simulink model "sampleModel1722_2"  (R2023a)
settings: Solver=VariableStepAuto  StartTime=0.0  StopTime=10.0  RelTol=1e-3
libraries: hdlsllib x5, simulink x1
settings Model: Creator=user1  LastModifiedBy=user1

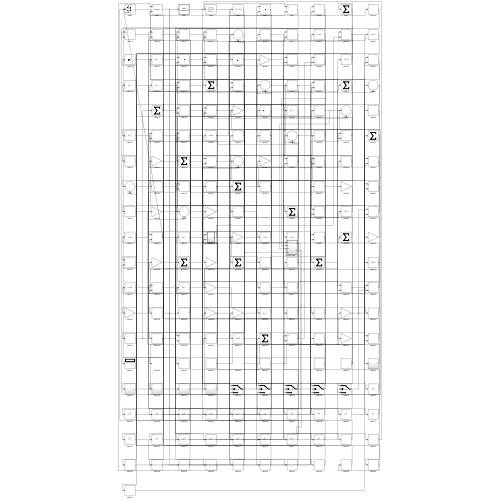
[thumbnail: Simulink's stored preview of the top-level diagram]
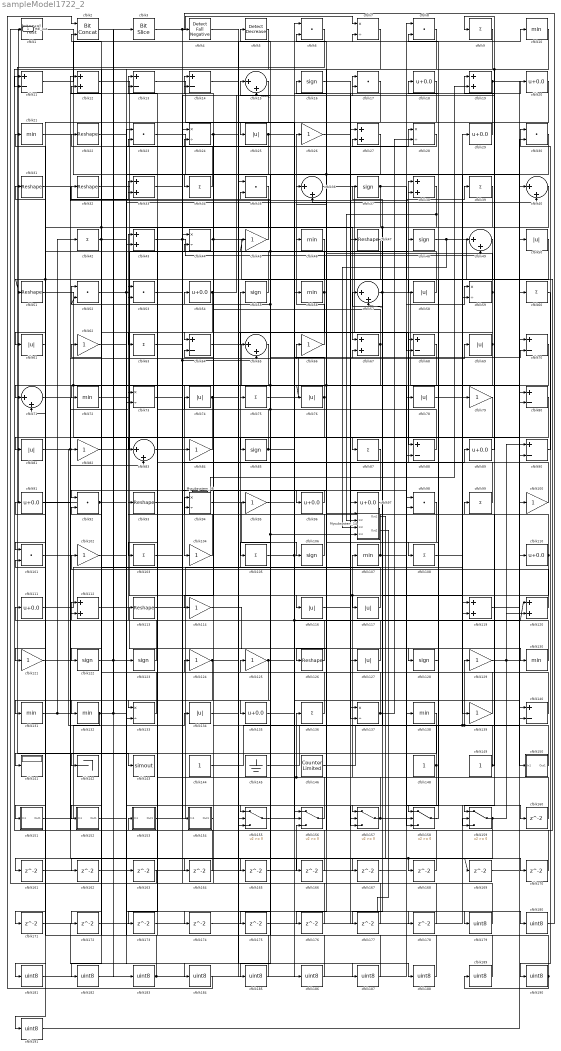
== system sampleModel1722_2 ==
  Mysubsystem_14 : Subsystem  TreatAsAtomicUnit=on  RTWFcnName=Mysubsystem_14
      settings: RTWFcnNameOpts=User specified  RTWFileNameOpts=Use function name
  Mysubsystem_36 : Subsystem  TreatAsAtomicUnit=on  RTWFcnName=Mysubsystem_36
      settings: RTWFcnNameOpts=User specified  RTWFileNameOpts=Use function name
  cfblk1 : hdlsllib/Logic and Bit Operations/Interval Test  IntervalClosedRight=on  uplimit=0.5  IntervalClosedLeft=on  lowlimit=-0.5  OutDataTypeStr=uint8
  cfblk{10,21,46,56,72,107,130..132,138} (10 alike) : MinMax  OutDataTypeStr=uint8
  cfblk{26,45,62,66,79,82,84,95,100,102,104,114,121,124..125,129,139} (17 alike) : Gain  OutDataTypeStr=uint8
  cfblk{6,8,17,23,30,35,52..53,92,98,101} (11 alike) : DotProduct  OutDataTypeStr=uint8
  cfblk{9,34,39,42,60,63,75,87,99,103,105,108,136} (13 alike) : Sum  Inputs=+  OutDataTypeStr=uint8
  cfblk{16,37,48,55,85,106,122..123,128} (9 alike) : Signum
  cfblk{11,13..14,64,68,70,80,88,90,140} (10 alike) : Sum  Inputs=+-  OutDataTypeStr=uint8
  cfblk{18,20,29,54,89,91,96..97,110..111,135} (11 alike) : Bias  Bias=0.0  SaturateOnIntegerOverflow=off
  cfblk{12,19,27,33,38,43,67,112,119..120} (10 alike) : Sum  OutDataTypeStr=uint8
  cfblk{22,31..32,47,51,93,113,126} (8 alike) : Reshape
  cfblk{25,50,58,61,69,74,76,78,81,116..117,127,134} (13 alike) : Abs  OutDataTypeStr=uint8  SaturateOnIntegerOverflow=off
  cfblk{7,24,28,44,59,73,94,133,137} (9 alike) : Product  Inputs=*/  OutDataTypeStr=uint8  RndMeth=Zero  SaturateOnIntegerOverflow=on
  cfblk141 : Display
  cfblk142 : Terminator
  cfblk143 : ToWorkspace  VariableName=simout  SaveFormat=Timeseries  SampleTime=-1
  cfblk144 : Constant  OutDataTypeStr=uint8  SampleTime=-1
  cfblk145 : Ground
  cfblk146 : hdlsllib/Sources/Counter Limited  uplimit=7  tsamp=-1
  cfblk148 : Constant  OutDataTypeStr=uint8  SampleTime=-1
  cfblk149 : Constant  OutDataTypeStr=uint8  SampleTime=-1
  cfblk{15,36,40,49,57,65,71,83} (8 alike) : Sum  Inputs=|++  OutDataTypeStr=uint8
  cfblk150 : Subsystem
      settings: LibrarySourceBlock=|
      | hdlsllib/Ports &
      | Subsystems/Subsystem
  cfblk151 : Subsystem
      settings: LibrarySourceBlock=|
      | hdlsllib/Ports &
      | Subsystems/Subsystem
  cfblk152 : Subsystem
      settings: LibrarySourceBlock=|
      | hdlsllib/Ports &
      | Subsystems/Subsystem
  cfblk153 : Subsystem
      settings: LibrarySourceBlock=|
      | hdlsllib/Ports &
      | Subsystems/Subsystem
  cfblk154 : Subsystem
      settings: LibrarySourceBlock=|
      | hdlsllib/Ports &
      | Subsystems/Subsystem
  cfblk{155..159} (5 alike) : Switch  OutDataTypeStr=uint8  SaturateOnIntegerOverflow=off  InputSameDT=off
  cfblk{160..178} (19 alike) : Delay  SampleTime=1
  cfblk{179..191} (13 alike) : DataTypeConversion  OutDataTypeStr=uint8  SaturateOnIntegerOverflow=off  RndMeth=Floor
  cfblk2 : hdlsllib/Logic and Bit Operations/Bit Concat  numInputs=2
  cfblk3 : hdlsllib/Logic and Bit Operations/Bit Slice  lidx=7  ridx=0
  cfblk4 : hdlsllib/Logic and Bit Operations/Detect Fall Negative  vinit=0  OutDataTypeStr=uint8
  cfblk5 : simulink/Logic and Bit Operations/Detect Decrease  vinit=0.0  OutDataTypeStr=uint8
      settings: LibrarySourceBlock=|
      | hdlsllib/Logic and Bit
      | Operations/Detect
      | Decrease
  Hdl_out : Outport  OutDataTypeStr=uint8
  wires:
  cfblk131/1 -> cfblk42/1, cfblk33/2
  cfblk100/1 -> cfblk38/1
  cfblk9/1 -> cfblk132/1
  cfblk132/1 -> cfblk3/1, cfblk159/3, cfblk82/1
  cfblk6/1 -> cfblk143/1
  cfblk66/1 -> cfblk26/1
  cfblk65/1 -> cfblk104/1
  cfblk157/1 -> cfblk107/1, cfblk39/1
  cfblk120/1 -> cfblk102/1
  cfblk12/1 -> cfblk116/1
  cfblk122/1 -> cfblk163/1, cfblk180/1
  cfblk113/1 -> cfblk55/1
  cfblk96/1 -> cfblk92/1
  cfblk103/1 -> cfblk117/1, cfblk119/2
  cfblk54/1 -> cfblk9/1, cfblk142/1
  cfblk98/1 -> cfblk126/1
  cfblk159/1 -> cfblk90/1, cfblk191/1
  cfblk107/1 -> cfblk75/1, cfblk59/1
  cfblk25/1 -> cfblk34/1, cfblk58/1
  cfblk133/1 -> cfblk92/2
  cfblk111/1 -> cfblk84/1
  cfblk123/1 -> cfblk43/1
  cfblk2/1 -> cfblk183/1
  cfblk32/1 -> cfblk67/1
  cfblk48/1 -> Mysubsystem_14/3(In3), cfblk153/1(In1)
  cfblk39/1 -> cfblk103/1, cfblk57/2
  cfblk117/1 -> cfblk52/1
  cfblk51/1 -> cfblk87/1, cfblk97/1
  cfblk112/1 -> cfblk130/1
  cfblk44/1 -> cfblk150/1(In1), cfblk14/1
  cfblk74/1 -> cfblk7/2, cfblk182/1
  cfblk85/1 -> cfblk74/1, cfblk157/3
  cfblk130/1 -> cfblk46/1
  cfblk19/1 -> cfblk140/1, cfblk81/1
  cfblk69/1 -> cfblk101/1, cfblk63/1
  cfblk42/1 -> cfblk28/1, cfblk12/2
  cfblk30/1 -> cfblk85/1
  cfblk153/1(Out1) -> cfblk29/1
  cfblk68/1 -> cfblk76/1, cfblk166/1
  cfblk47/1 -> cfblk133/1
  cfblk36/1 -> cfblk88/1
  cfblk145/1 -> cfblk129/1, cfblk90/2, cfblk79/1
  cfblk126/1 -> cfblk111/1
  cfblk92/1 -> cfblk123/1, Hdl_out/1
  cfblk27/1 -> Mysubsystem_14/1(In1), cfblk133/2
  cfblk99/1 -> cfblk32/1
  cfblk79/1 -> cfblk158/1
  cfblk83/1 -> cfblk66/1
  cfblk13/1 -> cfblk156/1
  cfblk82/1 -> cfblk48/1
  cfblk91/1 -> cfblk69/1
  cfblk140/1 -> cfblk13/1
  cfblk97/1 -> cfblk37/1
  cfblk11/1 -> cfblk10/1
  cfblk49/1 -> cfblk108/1
  cfblk20/1 -> cfblk122/1
  cfblk106/1 -> cfblk5/1
  cfblk110/1 -> cfblk93/1, cfblk167/1
  cfblk15/1 -> cfblk51/1, cfblk151/1(In1)
  cfblk35/1 -> cfblk171/1, cfblk172/1
  cfblk73/1 -> cfblk17/1, cfblk65/2
  cfblk67/1 -> cfblk72/1, cfblk24/2
  cfblk139/1 -> cfblk112/1
  cfblk144/1 -> cfblk78/1
  cfblk108/1 -> cfblk119/1
  cfblk56/1 -> cfblk64/1, cfblk35/2
  cfblk37/1 -> cfblk135/1, cfblk59/2
  cfblk146/1 -> cfblk40/1
  cfblk29/1 -> cfblk25/1
  cfblk137/1 -> cfblk54/1, cfblk28/2
  cfblk81/1 -> cfblk168/1, cfblk169/1, cfblk14/2
  cfblk116/1 -> cfblk20/1
  cfblk128/1 -> cfblk18/1
  cfblk78/1 -> cfblk49/1
  cfblk72/1 -> cfblk6/1
  cfblk31/1 -> cfblk38/2
  cfblk23/1 -> cfblk80/1
  cfblk84/1 -> cfblk83/1
  cfblk57/1 -> cfblk100/1, cfblk177/1
  cfblk59/1 -> cfblk6/2, cfblk176/1
  cfblk94/1 -> cfblk106/1
  cfblk33/1 -> cfblk154/1(In1)
  cfblk52/1 -> cfblk110/1, cfblk155/2
  cfblk10/1 -> cfblk43/2, cfblk159/1
  cfblk26/1 -> cfblk47/1
  cfblk16/1 -> cfblk127/1
  cfblk129/1 -> cfblk70/1, cfblk120/2
  cfblk71/1 -> cfblk83/2
  cfblk76/1 -> cfblk45/1, cfblk22/1, cfblk52/2, cfblk175/1
  cfblk104/1 -> cfblk53/1
  cfblk75/1 -> cfblk67/2
  cfblk89/1 -> cfblk19/1
  cfblk124/1 -> cfblk152/1(In1), cfblk187/1
  cfblk43/1 -> cfblk49/2, cfblk160/1
  cfblk121/1 -> cfblk73/1
  cfblk90/1 -> cfblk30/1
  cfblk156/1 -> cfblk136/1, cfblk113/1
  cfblk80/1 -> cfblk121/1
  cfblk21/1 -> cfblk80/2
  cfblk151/1(Out1) -> cfblk134/1
  cfblk45/1 -> cfblk33/1
  cfblk155/1 -> cfblk70/2
  cfblk119/1 -> cfblk50/1
  cfblk18/1 -> cfblk71/1
  cfblk7/1 -> cfblk73/2
  cfblk64/1 -> cfblk158/2
  cfblk46/1 -> cfblk105/1
  cfblk1/1 -> cfblk139/1
  cfblk63/1 -> cfblk98/2
  cfblk127/1 -> cfblk94/1
  cfblk136/1 -> cfblk125/1
  cfblk105/1 -> cfblk56/1, cfblk140/2
  cfblk60/1 -> cfblk190/1
  cfblk70/1 -> cfblk71/2, cfblk185/1, cfblk96/1
  cfblk50/1 -> cfblk61/1
  cfblk114/1 -> cfblk156/2
  cfblk148/1 -> cfblk158/3, cfblk44/2
  cfblk88/1 -> cfblk15/1, cfblk53/2
  cfblk28/1 -> cfblk27/2
  cfblk154/1(Out1) -> cfblk124/1
  cfblk158/1 -> cfblk8/2
  cfblk24/1 -> cfblk114/1, cfblk68/2
  cfblk38/1 -> Mysubsystem_14/2(In2), cfblk173/1
  cfblk150/1(Out1) -> Mysubsystem_14/4(In4), cfblk15/2
  cfblk58/1 -> cfblk16/1
  cfblk134/1 -> cfblk68/1
  cfblk87/1 -> cfblk137/2
  cfblk93/1 -> cfblk89/1
  cfblk135/1 -> cfblk157/1
  cfblk152/1(Out1) -> cfblk40/2
  cfblk5/1 -> cfblk11/2
  cfblk34/1 -> cfblk13/2
  cfblk3/1 -> cfblk7/1, cfblk155/1
  cfblk149/1 -> cfblk99/1, cfblk57/1
  cfblk125/1 -> cfblk120/1, cfblk17/2, cfblk131/1
  cfblk55/1 -> cfblk21/1
  cfblk40/1 -> cfblk65/1
  cfblk17/1 -> cfblk141/1
  cfblk53/1 -> cfblk128/1
  cfblk8/1 -> cfblk36/2
  cfblk160/1 -> cfblk64/2
  cfblk61/1 -> cfblk161/1
  cfblk161/1 -> cfblk88/2
  cfblk162/1 -> cfblk27/1
  cfblk163/1 -> cfblk1/1
  cfblk101/1 -> cfblk164/1
  cfblk164/1 -> cfblk12/1
  cfblk102/1 -> cfblk165/1
  cfblk165/1 -> cfblk156/3
  cfblk166/1 -> cfblk24/1
  cfblk167/1 -> cfblk8/1
  cfblk168/1 -> cfblk36/1
  cfblk169/1 -> cfblk30/2
  cfblk14/1 -> cfblk170/1
  cfblk170/1 -> cfblk11/1
  cfblk172/1 -> cfblk159/2
  cfblk173/1 -> cfblk155/3
  cfblk22/1 -> cfblk174/1
  cfblk174/1 -> cfblk137/1
  cfblk175/1 -> cfblk157/2
  cfblk176/1 -> cfblk112/2
  cfblk177/1 -> cfblk94/2
  cfblk178/1 -> cfblk44/1
  cfblk4/1 -> cfblk179/1
  cfblk179/1 -> cfblk91/1
  cfblk180/1 -> cfblk4/1
  cfblk138/1 -> cfblk181/1
  cfblk181/1 -> cfblk98/1
  cfblk182/1 -> cfblk138/1
  cfblk183/1 -> cfblk31/1, cfblk35/1
  cfblk171/1 -> cfblk184/1
  cfblk184/1 -> cfblk2/1
  cfblk185/1 -> cfblk2/2
  cfblk95/1 -> cfblk186/1
  cfblk186/1 -> cfblk23/2
  cfblk187/1 -> cfblk95/1
  cfblk62/1 -> cfblk188/1
  cfblk188/1 -> cfblk23/1
  cfblk189/1 -> cfblk62/1
  cfblk190/1 -> cfblk189/1, cfblk101/2
  cfblk191/1 -> cfblk60/1
  Mysubsystem_14/1(Out1) -> cfblk162/1
  Mysubsystem_14/2(Out2) -> cfblk178/1
  Mysubsystem_36/1(Out1) -> cfblk19/2

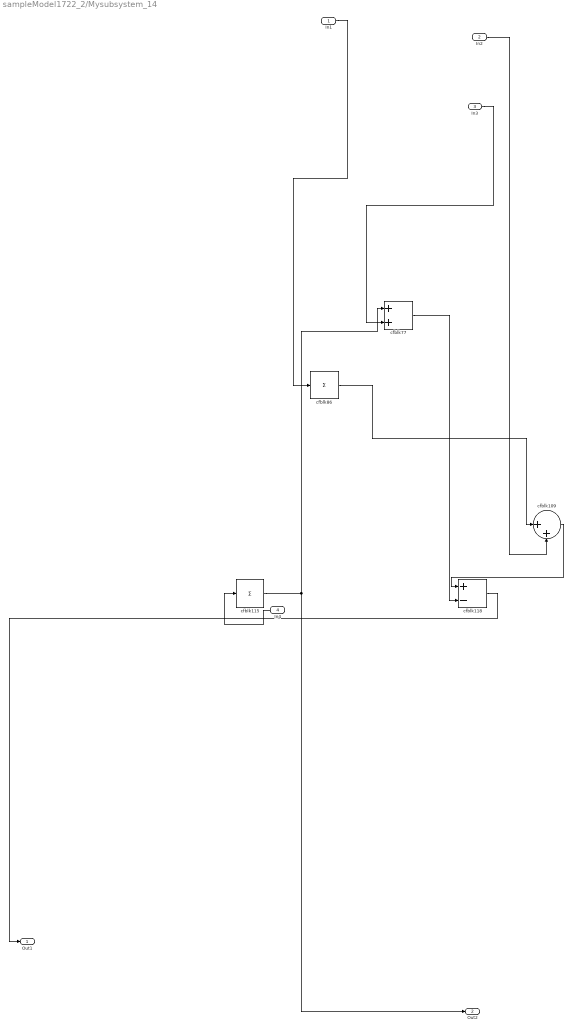
== system sampleModel1722_2/Mysubsystem_14 ==
  In1 : Inport
  In2 : Inport  Port=2
  In3 : Inport  Port=3
  In4 : Inport  Port=4
  cfblk109 : Sum  Inputs=|++
  cfblk115 : Sum  Inputs=+
  cfblk118 : Sum  Inputs=+-
  cfblk77 : Sum
  cfblk86 : Sum  Inputs=+
  Out1 : Outport
  Out2 : Outport  Port=2
  wires:
  cfblk109/1 -> cfblk118/1
  cfblk118/1 -> Out1/1
  cfblk86/1 -> cfblk109/1
  cfblk115/1 -> Out2/1, cfblk77/1
  In2/1 -> cfblk109/2
  cfblk77/1 -> cfblk118/2
  In4/1 -> cfblk115/1
  In1/1 -> cfblk86/1
  In3/1 -> cfblk77/2

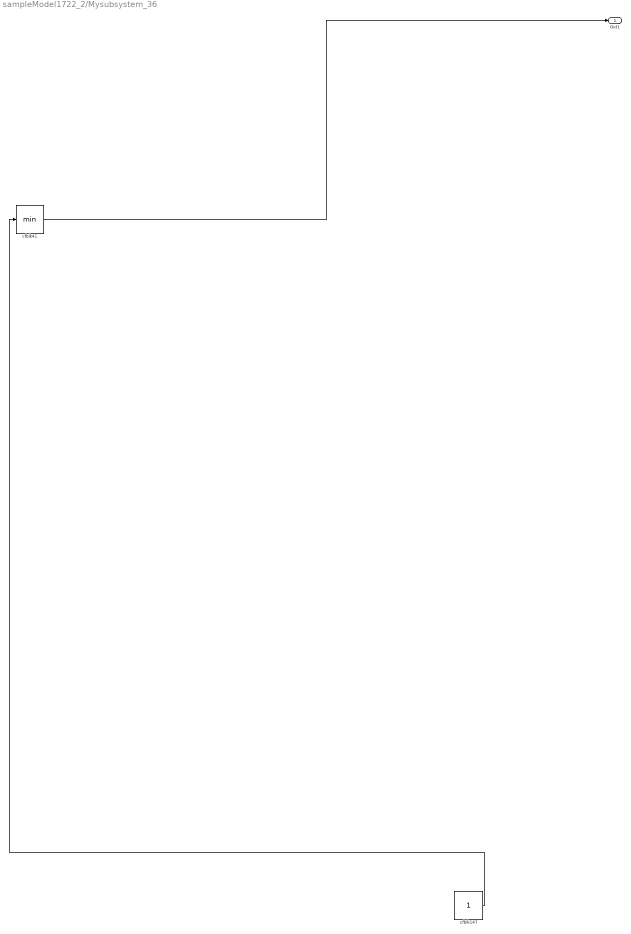
== system sampleModel1722_2/Mysubsystem_36 ==
  cfblk147 : Constant  SampleTime=-1
  cfblk41 : MinMax
  Out1 : Outport
  wires:
  cfblk147/1 -> cfblk41/1
  cfblk41/1 -> Out1/1

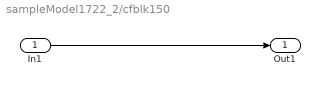
== system sampleModel1722_2/cfblk150 ==
  In1 : Inport
  Out1 : Outport
  wires:
  In1/1 -> Out1/1

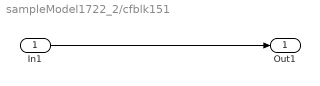
== system sampleModel1722_2/cfblk151 ==
  In1 : Inport
  Out1 : Outport
  wires:
  In1/1 -> Out1/1

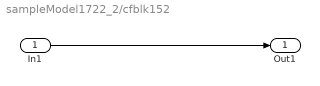
== system sampleModel1722_2/cfblk152 ==
  In1 : Inport
  Out1 : Outport
  wires:
  In1/1 -> Out1/1

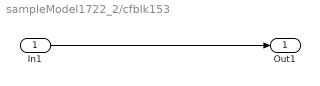
== system sampleModel1722_2/cfblk153 ==
  In1 : Inport
  Out1 : Outport
  wires:
  In1/1 -> Out1/1

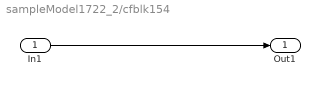
== system sampleModel1722_2/cfblk154 ==
  In1 : Inport
  Out1 : Outport
  wires:
  In1/1 -> Out1/1
